simulink model "CruiseState_tmp"  (Simulink 8.4)
settings: Solver=ode45  StartTime=0.0  StopTime=10.0  RelTol=1e-3
settings Model: Creator=bourbouh  LastModifiedBy=hbourbou  CovSFcnEnable=on
settings DataIOCC: LimitDataPoints=off  SaveFormat=StructureWithTime  SignalLoggingSaveFormat=Dataset
settings OptimizationCC: ExpressionDepthLimit=128
settings DebuggingCC: UnderspecifiedInitializationDetection=Simplified  MergeDetectMultiDrivingBlocksExec=error  SolverPrmCheckMsg=none  FcnCallInpInsideContextMsg=EnableAllAsError  FrameProcessingCompatibilityMsg=error  StateNameClashWarn=none
settings HardwareCC: ProdBitPerPointer=64  ProdLargestAtomicFloat=Float  ProdIntDivRoundTo=Zero  ProdEndianess=LittleEndian  ProdHWDeviceType=Specified
settings ModelReferenceCC: PropagateSignalLabelsOutOfModel=on
settings GRTTargetCC: CombineOutputUpdateFcns=on  GRTInterface=off

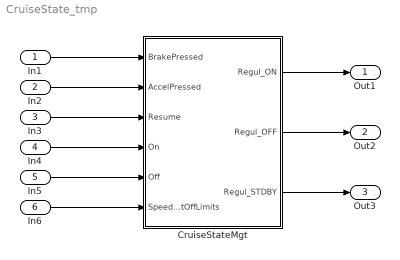
== system CruiseState_tmp ==
  In1 : Inport
  In2 : Inport  Port=2
  In3 : Inport  Port=3
  In4 : Inport  Port=4
  In5 : Inport  Port=5
  In6 : Inport  Port=6
  CruiseStateMgt : Stateflow chart  TreatAsAtomicUnit=on
      settings: PermitHierarchicalResolution=ParametersOnly
  Out1 : Outport
  Out2 : Outport  Port=2
  Out3 : Outport  Port=3
  wires:
  In1/1 -> CruiseStateMgt/1(BrakePressed)
  In2/1 -> CruiseStateMgt/2(AccelPressed)
  In3/1 -> CruiseStateMgt/3(Resume)
  In4/1 -> CruiseStateMgt/4(On)
  In5/1 -> CruiseStateMgt/5(Off)
  In6/1 -> CruiseStateMgt/6(SpeedOutOffLimits)
  CruiseStateMgt/1(Regul_ON) -> Out1/1
  CruiseStateMgt/2(Regul_OFF) -> Out2/1
  CruiseStateMgt/3(Regul_STDBY) -> Out3/1

== stateflow chart CruiseStateMgt ==
  settings: updateMethod=DISCRETE
  state Disabled
    entry:
    Regul_OFF = 1;
    Regul_ON = 0;
    Regul_STDBY = 0
  state Enabled
    state Interrupted
      entry:
      Regul_OFF = 1;
      Regul_ON = 0;
      Regul_STDBY = 1
    state Regulation
      state On
        entry:
        Regul_OFF = 0;
        Regul_ON = 1;
        Regul_STDBY = 0
      state StandBy
        entry:
        Regul_OFF = 0;
        Regul_ON = 0;
        Regul_STDBY = 1
      (default) -> (junction 9)
      (junction 9) -> StandBy [order 1] : [AccelPressed  | SpeedOutOffLimits ]
      (junction 9) -> On [order 2]
      On -> StandBy : [AccelPressed  | SpeedOutOffLimits ]
      StandBy -> On : [~AccelPressed & ~SpeedOutOffLimits]
    (default) -> (junction 15)
    (junction 15) -> Regulation [order 2]
    (junction 15) -> Interrupted [order 1] : [BrakePressed]
    Regulation -> Interrupted : [BrakePressed]
    Interrupted -> Regulation : [Resume & ~BrakePressed]
  (default) -> (junction 30)
  (junction 30) -> Disabled [order 2]
  (junction 30) -> Enabled [order 1] : [On]
  Disabled -> Enabled : [On]
  Enabled -> Disabled : [Off]
  data: BrakePressed input boolean; AccelPressed input boolean; Resume input boolean; On input boolean; Off input boolean; SpeedOutOffLimits input boolean; Regul_ON output boolean; Regul_OFF output boolean; Regul_STDBY output boolean
